simulink model "IEEE_3SG_9bus"  (R2023b)
settings: Solver=ode8  StartTime=0.0  StopTime=20  RelTol=1e-4  EnableMultiTasking=on
PreLoadFcn:
  | ct = 1.083
undefined symbols (not defined in the file): D1, Delta
libraries: spsThreePhaseVIMeasurementLib x12, spsLoadFlowBusLib x9, spsThreePhasePISectionLineLib x6, jailib x3, spsSynchronousMachinepuStandardLib x3, spsThreePhaseTransformerTwoWindingsLib x3, spsDC1AExcitationSystemLib x3, spsPowerPositiveSequenceLib x3, spsThreePhaseBreakerLib x2, spsSequenceAnalyzerLib x1, spsThreePhaseFaultLib x1, spspowerguiLib x1
settings Model: SimulationMode=accelerator  Creator=jp536285  LastModifiedBy=Administrator
settings SolverCC: AlgebraicLoopSolver=TrustRegion  AutoInsertRateTranBlk=on
settings DataIOCC: SaveFormat=Array  SaveOutput=off  SaveTime=off  ReturnWorkspaceOutputs=off
settings OptimizationCC: LifeSpan=inf
settings DebuggingCC: UnderspecifiedInitializationDetection=Classic  MergeDetectMultiDrivingBlocksExec=none  SolverPrmCheckMsg=warning  StateNameClashWarn=warning  SFUnexpectedBacktrackingDiag=warning  SFNoUnconditionalDefaultTransitionDiag=warning  SFExecutionAtInitializationDiag=none  ArithmeticOperatorsInVariantConditions=warning
settings HardwareCC: ProdBitPerPointer=32  ProdBitPerSizeT=32  ProdBitPerPtrDiffT=32  ProdLargestAtomicFloat=None  ProdIntDivRoundTo=Undefined  ProdEndianess=Unspecified  ProdWordSize=32  ProdHWDeviceType=32-bit Generic
settings ModelReferenceCC: PropagateSignalLabelsOutOfModel=off
settings SFSimCC: SimUseLocalCustomCode=off  CustomCodeUndefinedFunction=UseInterfaceOnly
settings RTWCC: RTWUseLocalCustomCode=off
settings CodeAppCC: StateflowObjectComments=on
settings GRTTargetCC: TargetLangStandard=C89/C90 (ANSI)
settings ConfigComp: CovMetricSettings=dw  CovSaveCumulativeToWorkspaceVar=on  CovSaveSingleToWorkspaceVar=on  CovExternalEMLEnable=off
settings SimscapeCC: SimscapeNormalizeSystem=off

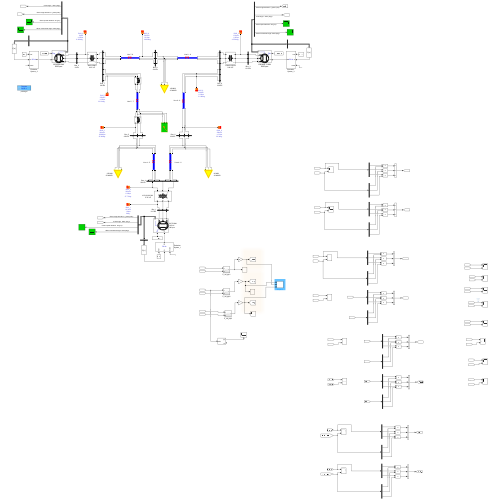
[thumbnail: Simulink's stored preview of the top-level diagram]
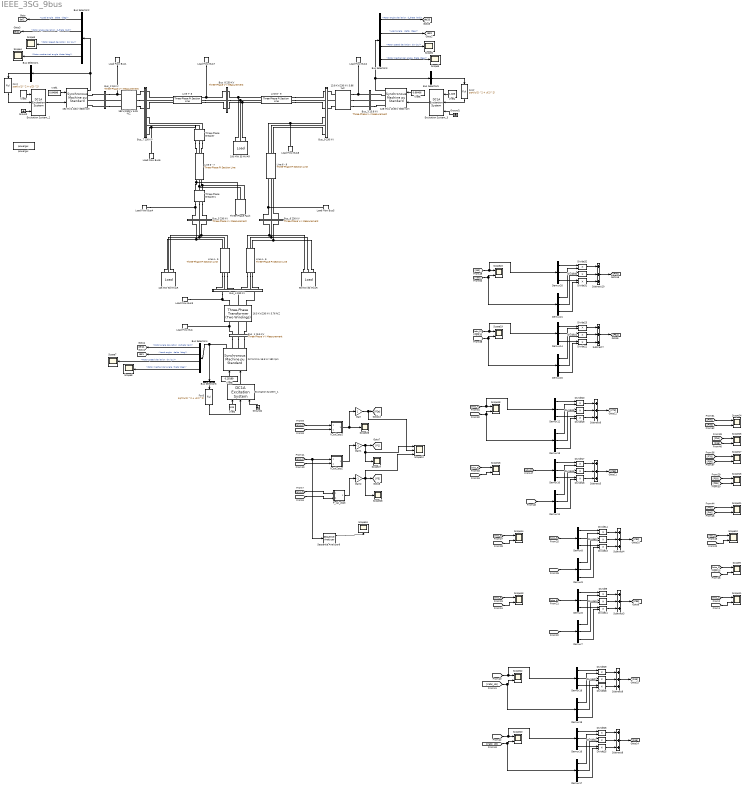
== system IEEE_3SG_9bus ==
  " Line 4 - 6" : spsThreePhasePISectionLineLib/Three-Phase PI Section Line  LConnTagsString=a|b|c  RConnTagsString=A|B|C  Length=100  Frequency=60  Resistances=[ 0.08993 0.224825]  Inductances="[ 1.29e-3  3.22e-3]"  Capacitances=[7.922e-9 4.74e-9]  mask(Three-Phase PI Section Line){}
      mask Display:
      | % This is a new mask on top of the base mask.
      | % Use "View base mask" link below to see the base mask.
      | patch([0.0 0.0 1 1 0.0 0.0 ],[0.4 0.7 0.7 0.4 0.4 0.7],[0 0 1]);
      | patch([0.4 0.4 0.42 0.42],[0.4 0.75 0.75 0.4],[1 0 0]);
      | patch([0.38 0.38 0.57 0.57],[0.7 0.75 0.75 0.7],[1 0 0]);
      | patch([0.53 0.53 0.55 0.55],[0.4 0.75 0.75 0.4],[1 0 0]);
  " Line 6 - 9" : spsThreePhasePISectionLineLib/Three-Phase PI Section Line  LConnTagsString=a|b|c  RConnTagsString=A|B|C  Length=100  Frequency=60  Resistances=[ 0.20631 0.5157]  Inductances="[ 2.38e-3  6.09e-3]"  Capacitances=[17.95e-9 10.55e-9]  mask(Three-Phase PI Section Line){}
      mask Display:
      | % This is a new mask on top of the base mask.
      | % Use "View base mask" link below to see the base mask.
      | patch([0.0 0.0 1 1 0.0 0.0 ],[0.4 0.7 0.7 0.4 0.4 0.7],[0 0 1]);
      | patch([0.4 0.4 0.42 0.42],[0.4 0.75 0.75 0.4],[1 0 0]);
      | patch([0.38 0.38 0.57 0.57],[0.7 0.75 0.75 0.7],[1 0 0]);
      | patch([0.53 0.53 0.55 0.55],[0.4 0.75 0.75 0.4],[1 0 0]);
  100 MW 35 MVAR : jailib/Load  SystemSampleTime=-1  VariantActivationTime=update diagram  AllowFlexibleInterface=on  Latency=0  AutoFrameSizeCalculation=off
      link override Three-Phase Parallel RLC Load: NominalVoltage=(230000)*1.01602  ActivePower=100e6  InductivePower=35e6  LoadType=constant PQ
      settings: SourceProductName=Power Library
  125 MW 50 MVAR : jailib/Load  SystemSampleTime=-1  VariantActivationTime=update diagram  AllowFlexibleInterface=on  Latency=0  AutoFrameSizeCalculation=off
      link override Three-Phase Parallel RLC Load: NominalVoltage=(230000)*0.996183  ActivePower=125e6  InductivePower=50e6  LoadType=constant PQ
      settings: SourceProductName=Power Library
  128 MVA 13.8kV 3600 rpm : spsSynchronousMachinepuStandardLib/Synchronous Machine pu Standard  PresetModel=No  MechanicalLoad=Mechanical power Pm  ShowDetailedParameters=on  RotorType=Round  Units=per unit standard parameters  MeasurementBus=off  NominalParameters="[ 128e6  13.8e3   60 ]"  Reactances1=[ 1.68, 0.23206, 0.19, 1.61, 0.23206, 0.19, 0.314]  Reactances2="[ 1.305, 0.296, 0.252, 0.474,  0.243,  0.18 ]"  dAxisTimeConstants=Open-circuit  qAxisTimeConstants=Open-circuit  TimeConstants1="[ 4.4849  0.0681  0.1  ]"  TimeConstants2=[ 5.89, 0.001,0.6, 0.001 ]  TimeConstants3="[  4.49  0.0681  0.0513  ]"  TimeConstants4=[ 8.0, 0.03, 0.3371, 0.0295 ]  TimeConstants5=[ 1.01, 0.053, 0.1 ]  TimeConstants6=[ 1.3201, 0.023, 1.0, 0.07 ]  TimeConstants7="[  1.01  0.053  0.051266  ]"  TimeConstants8=[ 1.3201, 0.0231, 0.3371, 0.0295 ]  StatorResistance=1e-7  Mechanical="[ 2.35  0 1 ]"  PolePairs=1  InitialConditions=[0 -36.0034 0.653061 0.653061 0.653061 11.785 -108.215 131.785 1.40359]  SetSaturation=off  Saturation=[0.6404,0.7127,0.8441,0.9214,0.9956,1.082,1.19,1.316,1.457;0.7,0.7698,0.8872,0.9466,0.9969,1.046,1.1,1.151,1.201]  LoadFlowParameters=[1 85000000 0 0 0]  TsPowergui=0  TsBlock=-1  IterativeModel=Trapezoidal non iterative  IterativeDiscreteModel=Trapezoidal non iterative  BusType=PV  Pref=85000000  Qref=0  Qmin=-Inf  Qmax=Inf  PLF=0  QLF=0
  13.8 KV/230 KV 5.86 %Z : spsThreePhaseTransformerTwoWindingsLib/Three-Phase Transformer (Two Windings)  Winding1Connection=Delta (D1)  Winding2Connection=Yg  CoreType=Three single-phase transformers  SetSaturation=off  Hysteresis=off  DataFile='hysteresis'  SetInitialFlux=off  Measurements=None  UNITS=pu  NominalPower=[ 100e6 , 60 ]  Winding1=[ 13.8e3 , 1e-6 , 0 ]  Winding2=[ 230e3 , 1e-6, 0.0586 ]  Rm=500  Lm=500  L0=0.5  Saturation=[ 0,0 ; 0.0024,1.2 ; 1.0,1.52 ]  InitialFluxes=[ 0.8 , -0.8 , 0.7 ]  BreakLoop=off  DiscreteSolver=Trapezoidal iterative  DataType=off  TransfoNumber=1
  "16.5 KV/230 KV 5.76 %Z     " : spsThreePhaseTransformerTwoWindingsLib/Three-Phase Transformer (Two Windings)  Winding1Connection=Delta (D1)  Winding2Connection=Yg  CoreType=Three single-phase transformers  SetSaturation=off  Hysteresis=off  DataFile='hysteresis'  SetInitialFlux=off  Measurements=None  UNITS=pu  NominalPower=[ 100e6 , 60 ]  Winding1=[ 16.5e3 , 1e-6, 0 ]  Winding2=[ 230e3 ,1e-6, 0.0576 ]  Rm=500  Lm=500  L0=0.5  Saturation=[ 0,0 ; 0.0024,1.2 ; 1.0,1.52 ]  InitialFluxes=[ 0.8 , -0.8 , 0.7 ]  BreakLoop=off  DiscreteSolver=Trapezoidal iterative  DataType=off  TransfoNumber=1
  18KV/230KV 6.25 %Z : spsThreePhaseTransformerTwoWindingsLib/Three-Phase Transformer (Two Windings)  Winding1Connection=Delta (D1)  Winding2Connection=Yg  CoreType=Three single-phase transformers  SetSaturation=off  Hysteresis=off  DataFile='hysteresis'  SetInitialFlux=off  Measurements=None  UNITS=pu  NominalPower=[ 100e6 , 60 ]  Winding1=[ 18e3 , 1e-6 , 0]  Winding2=[ 230e3 , 1e-6, 0.0625 ]  Rm=500  Lm=500  L0=0.5  Saturation=[ 0,0 ; 0.0024,1.2 ; 1.0,1.52 ]  InitialFluxes=[ 0.8 , -0.8 , 0.7 ]  BreakLoop=off  DiscreteSolver=Trapezoidal iterative  DataType=off  TransfoNumber=1
  192 MVA 18kV 3600 rpm : spsSynchronousMachinepuStandardLib/Synchronous Machine pu Standard  PresetModel=No  MechanicalLoad=Mechanical power Pm  ShowDetailedParameters=on  RotorType=Round  Units=per unit standard parameters  MeasurementBus=off  NominalParameters="[ 192e6  18e3   60 ]"  Reactances1=[ 1.72, 0.23, 0.1728,1.65, 0.23, 0.1728, 0.4224 ]  Reactances2="[ 1.305, 0.296, 0.252, 0.474,  0.243,  0.18 ]"  dAxisTimeConstants=Open-circuit  qAxisTimeConstants=Open-circuit  TimeConstants1="[ 4.4849  0.0681  0.1  ]"  TimeConstants2=[ 6, 0.001, 0.53, 0.001]  TimeConstants3="[  4.49  0.0681  0.0513  ]"  TimeConstants4=[ 8.0, 0.03, 0.3371, 0.0295 ]  TimeConstants5=[ 1.01, 0.053, 0.1 ]  TimeConstants6=[ 1.3201, 0.023, 1.0, 0.07 ]  TimeConstants7="[  1.01  0.053  0.051266  ]"  TimeConstants8=[ 1.3201, 0.0231, 0.3371, 0.0295 ]  StatorResistance=1e-7  Mechanical="[ 3.33  0 1 ]"  PolePairs=1  InitialConditions=[0 -29.1799 0.828949 0.828949 0.828949 6.81655 -113.183 126.817 1.78946]  SetSaturation=off  Saturation=[0.6404,0.7127,0.8441,0.9214,0.9956,1.082,1.19,1.316,1.457;0.7,0.7698,0.8872,0.9466,0.9969,1.046,1.1,1.151,1.201]  LoadFlowParameters=[1 163000000 0 0 0]  TsPowergui=0  TsBlock=-1  IterativeModel=Trapezoidal non iterative  IterativeDiscreteModel=Trapezoidal non iterative  BusType=PV  Pref=163000000  Qref=0  Qmin=-Inf  Qmax=Inf  PLF=0  QLF=0
  247.5 MVA 16.5 kV 180 rpm : spsSynchronousMachinepuStandardLib/Synchronous Machine pu Standard  PresetModel=No  MechanicalLoad=Mechanical power Pm  ShowDetailedParameters=on  RotorType=Salient-pole  Units=per unit standard parameters  MeasurementBus=off  NominalParameters="[ 247.5E6  16500   60 ]"  Reactances1=[ 31 32 33 34 35 36 37 ]  Reactances2=[ 0.361, 0.1504, 0.099, 0.2398, 0.099, 0.062 ]  dAxisTimeConstants=Open-circuit  qAxisTimeConstants=Open-circuit  TimeConstants1=[8.96 0.001 0.001]  TimeConstants2=[]  TimeConstants3=[]  TimeConstants4=[]  TimeConstants5=[ 1.01, 0.053, 0.31 ]  TimeConstants6=[]  TimeConstants7=[]  TimeConstants8=[]  StatorResistance=1e-7  Mechanical=[9.55 0 20]  PolePairs=20  InitialConditions=[0 -86.3839 0.299344 0.299344 0.299344 -20.3492 -140.349 99.6508 1.08182]  SetSaturation=off  Saturation=[0.6404,0.7127,0.8441,0.9214,0.9956,1.082,1.19,1.316,1.457;0.7,0.7698,0.8872,0.9466,0.9969,1.046,1.1,1.151,1.201]  LoadFlowParameters=[2 71000000 0 0]  TsPowergui=0  TsBlock=-1  IterativeModel=Trapezoidal non iterative  IterativeDiscreteModel=Trapezoidal non iterative  BusType=swing  Pref=150000000  Qref=0  Qmin=-Inf  Qmax=Inf  PLF=0  QLF=0
  90 MW 30 MVAR : jailib/Load  SystemSampleTime=-1  VariantActivationTime=update diagram  AllowFlexibleInterface=on  Latency=0  AutoFrameSizeCalculation=off
      link override Three-Phase Parallel RLC Load: NominalVoltage=(230000)*1.01315  ActivePower=90e6  InductivePower=30e6  LoadType=constant PQ
      settings: SourceProductName=Power Library
  Bus Selector1 : BusSelector  OutputSignals="dq0 components.Stator voltage  vq (pu),dq0 components.Stator voltage  vd (pu)"  OutputAsBus=on
  Bus Selector2 : BusSelector  OutputSignals="Load angle   delta  (deg),Mechanical.Rotor angle deviation  d_theta (rad),Mechanical.Rotor speed deviation  dw (pu),Mechanical.Rotor mechanical angle  theta (deg)"
  Bus Selector3 : BusSelector  OutputSignals="Mechanical.Rotor angle deviation  d_theta (rad),Load angle   delta  (deg),Mechanical.Rotor speed deviation  dw (pu),Mechanical.Rotor mechanical angle  theta (deg)"
  Bus Selector4 : BusSelector  OutputSignals="Mechanical.Rotor angle deviation  d_theta (rad),Load angle   delta  (deg),Mechanical.Rotor speed deviation  dw (pu),Mechanical.Rotor mechanical angle  theta (deg)"
  Bus Selector5 : BusSelector  OutputSignals="dq0 components.Stator voltage  vq (pu),dq0 components.Stator voltage  vd (pu)"  OutputAsBus=on
  Bus Selector6 : BusSelector  OutputSignals="dq0 components.Stator voltage  vq (pu),dq0 components.Stator voltage  vd (pu)"  OutputAsBus=on
  Bus_1 16.5 KV : spsThreePhaseVIMeasurementLib/Three-Phase V-I Measurement  VoltageMeasurement=phase-to-phase  SetLabelV=on  LabelV=Vabc_1  Vpu=off  VpuLL=off  CurrentMeasurement=yes  SetLabelI=on  LabelI=Iabc_1  Ipu=off  Pbase=100e6  Vbase=16.5e3  OutputType=Complex  PhasorSimulation=off  PSBequivalent=0
  Bus_2 18 KV : spsThreePhaseVIMeasurementLib/Three-Phase V-I Measurement  VoltageMeasurement=phase-to-phase  SetLabelV=on  LabelV=Vabc_2  Vpu=off  VpuLL=off  CurrentMeasurement=yes  SetLabelI=on  LabelI=Iabc_2  Ipu=off  Pbase=100e6  Vbase=18e3  OutputType=Complex  PhasorSimulation=off  PSBequivalent=0
  Bus_3 13.8 KV : spsThreePhaseVIMeasurementLib/Three-Phase V-I Measurement  VoltageMeasurement=phase-to-phase  SetLabelV=on  LabelV=Vabc_3  Vpu=off  VpuLL=off  CurrentMeasurement=yes  SetLabelI=on  LabelI=Iabc_3  Ipu=off  Pbase=100e6  Vbase=13.8e3  OutputType=Complex  PhasorSimulation=off  PSBequivalent=0
  Bus_4 230 KV : Subsystem
  Bus_5 230 KV : spsThreePhaseVIMeasurementLib/Three-Phase V-I Measurement  VoltageMeasurement=phase-to-ground  SetLabelV=on  LabelV=Vabc_5  Vpu=off  VpuLL=off  CurrentMeasurement=yes  SetLabelI=on  LabelI=Iabc_5  Ipu=off  Pbase=100e6  Vbase=230e3  OutputType=Complex  PhasorSimulation=off  PSBequivalent=0
  Bus_6 230 KV : spsThreePhaseVIMeasurementLib/Three-Phase V-I Measurement  VoltageMeasurement=phase-to-ground  SetLabelV=on  LabelV=Vabc_6  Vpu=off  VpuLL=off  CurrentMeasurement=yes  SetLabelI=on  LabelI=Iabc_6  Ipu=off  Pbase=100e6  Vbase=230e3  OutputType=Complex  PhasorSimulation=off  PSBequivalent=0
  Bus_7 230 KV : Subsystem
  Bus_8 230 KV : spsThreePhaseVIMeasurementLib/Three-Phase V-I Measurement  VoltageMeasurement=phase-to-ground  SetLabelV=on  LabelV=Vabc_8  Vpu=off  VpuLL=off  CurrentMeasurement=yes  SetLabelI=on  LabelI=Iabc_8  Ipu=off  Pbase=100e6  Vbase=230e3  OutputType=Complex  PhasorSimulation=off  PSBequivalent=0
  Bus_9 230 KV : Subsystem
  Demux{6..21} (16 alike) : Demux  Outputs=3
  Divide{9..32} (24 alike) : Product  Inputs=**
  Excitation System_2 : spsDC1AExcitationSystemLib/DC1A Excitation System  Tr=20e-3  KaTa=[20 0.2]  VRminmax=[ -4 4]  KfTf=[0.063 0.35]  TbTc=[0 0]  KeTe=[1 0.314]  Efd12=[3.1 2.3]  SeEfd12=[0.483 0.1394]  v0=[1.025 1.7895]  TsBlock=0
      settings: LibrarySourceBlock=|
      | sps_lib/Electrical Machines/Synchronous Machine Control/DC1A
      | Excitation System
  Excitation System_1 : spsDC1AExcitationSystemLib/DC1A Excitation System  Tr=20e-3  KaTa=[20 0.2]  VRminmax=[ -3 3]  KfTf=[0.063 0.35]  TbTc=[0 0]  KeTe=[1 0.314]  Efd12=[3.1 2.3]  SeEfd12=[0.483 0.1394]  v0=[1.04 1.0818]  TsBlock=0
      settings: LibrarySourceBlock=|
      | sps_lib/Electrical Machines/Synchronous Machine Control/DC1A
      | Excitation System
  Excitation System_3 : spsDC1AExcitationSystemLib/DC1A Excitation System  Tr=20e-3  KaTa=[20 0.2]  VRminmax=[-4 4]  KfTf=[0.063 0.35]  TbTc=[0 0]  KeTe=[1 0.314]  Efd12=[3.1 2.3]  SeEfd12=[0.483 0.1394]  v0=[1.025 1.4036]  TsBlock=0
      settings: LibrarySourceBlock=|
      | sps_lib/Electrical Machines/Synchronous Machine Control/DC1A
      | Excitation System
  Fcn1 : Fcn  Expr=sqrt(u(1)^2 + u(2)^2)
  Fcn2 : Fcn  Expr=sqrt(u(1)^2 + u(2)^2)
  Fcn3 : Fcn  Expr=sqrt(u(1)^2 + u(2)^2)
  Gain : Gain
  Gain1 : Gain  Gain=-1
  Gain2 : Gain  Gain=-1
  Ground : Ground
  Ground1 : Ground
  Ground2 : Ground
  "Line 4 - 5 " : spsThreePhasePISectionLineLib/Three-Phase PI Section Line  LConnTagsString=a|b|c  RConnTagsString=A|B|C  Length=100  Frequency=60  Resistances=[ 0.0529 0.13225]  Inductances="[ 1.192e-3  2.38e-3]"  Capacitances=[8.82e-9 5.188e-9]  mask(Three-Phase PI Section Line){}
      mask Display:
      | % This is a new mask on top of the base mask.
      | % Use "View base mask" link below to see the base mask.
      | patch([0.0 0.0 1 1 0.0 0.0 ],[0.4 0.7 0.7 0.4 0.4 0.7],[0 0 1]);
      | patch([0.4 0.4 0.42 0.42],[0.4 0.75 0.75 0.4],[1 0 0]);
      | patch([0.38 0.38 0.57 0.57],[0.7 0.75 0.75 0.7],[1 0 0]);
      | patch([0.53 0.53 0.55 0.55],[0.4 0.75 0.75 0.4],[1 0 0]);
  "Line 5 - 7 " : spsThreePhasePISectionLineLib/Three-Phase PI Section Line  LConnTagsString=a|b|c  RConnTagsString=A|B|C  Length=100  Frequency=60  Resistances=[ 0.16928 0.4232]  Inductances="[ 2.259e-3  5.64e-3]"  Capacitances=[15.34e-9 9.025e-9]  mask(Three-Phase PI Section Line){}
      mask Display:
      | % This is a new mask on top of the base mask.
      | % Use "View base mask" link below to see the base mask.
      | patch([0.0 0.0 1 1 0.0 0.0 ],[0.4 0.7 0.7 0.4 0.4 0.7],[0 0 1]);
      | patch([0.4 0.4 0.42 0.42],[0.4 0.75 0.75 0.4],[1 0 0]);
      | patch([0.38 0.38 0.57 0.57],[0.7 0.75 0.75 0.7],[1 0 0]);
      | patch([0.53 0.53 0.55 0.55],[0.4 0.75 0.75 0.4],[1 0 0]);
  Line 7- 8 : spsThreePhasePISectionLineLib/Three-Phase PI Section Line  LConnTagsString=a|b|c  RConnTagsString=A|B|C  Length=100  Frequency=60  Resistances=[0.044965 0.11241]  Inductances="[ 1.01e-3  2.02e-3]"  Capacitances=[7.471e-9 4.394e-9]  mask(Three-Phase PI Section Line){}
      mask Display:
      | % This is a new mask on top of the base mask.
      | % Use "View base mask" link below to see the base mask.
      | patch([0.0 0.0 1 1 0.0 0.0 ],[0.4 0.7 0.7 0.4 0.4 0.7],[0 0 1]);
      | patch([0.4 0.4 0.42 0.42],[0.4 0.75 0.75 0.4],[1 0 0]);
      | patch([0.38 0.38 0.57 0.57],[0.7 0.75 0.75 0.7],[1 0 0]);
      | patch([0.53 0.53 0.55 0.55],[0.4 0.75 0.75 0.4],[1 0 0]);
  Line 8 - 9 : spsThreePhasePISectionLineLib/Three-Phase PI Section Line  LConnTagsString=a|b|c  RConnTagsString=A|B|C  Length=100  Frequency=60  Resistances=[ 0.062951 0.15737]  Inductances="[ 1.414e-3  3.53e-3]"  Capacitances=[10.47e-9 6.15e-9]  mask(Three-Phase PI Section Line){}
      mask Display:
      | % This is a new mask on top of the base mask.
      | % Use "View base mask" link below to see the base mask.
      | patch([0.0 0.0 1 1 0.0 0.0 ],[0.4 0.7 0.7 0.4 0.4 0.7],[0 0 1]);
      | patch([0.4 0.4 0.42 0.42],[0.4 0.75 0.75 0.4],[1 0 0]);
      | patch([0.38 0.38 0.57 0.57],[0.7 0.75 0.75 0.7],[1 0 0]);
      | patch([0.53 0.53 0.55 0.55],[0.4 0.75 0.75 0.4],[1 0 0]);
  Load Flow Bus : spsLoadFlowBusLib/Load Flow Bus  LConnTagsString=a  Phases=single  Connectors=on one side  ID=BUS_1  Vbase=16.5e3  Vref=1.04  Vangle=0  VLF=1.04  VLFb=1  VLFc=1  angleLF=0  angleLFb=0  angleLFc=0
      settings: AttributesFormatString=%<ID>\n%<Vbase>V\n%<VLF>pu\n%<angleLF>deg.
  Load Flow Bus1 : spsLoadFlowBusLib/Load Flow Bus  LConnTagsString=a  Phases=single  Connectors=on one side  ID=BUS_2  Vbase=18e3  Vref=1.025  Vangle=0  VLF=1.025  VLFb=1  VLFc=1  angleLF=9.166  angleLFb=0  angleLFc=0
      settings: AttributesFormatString=%<ID>\n%<Vbase>V\n%<VLF>pu\n%<angleLF>deg.
  Load Flow Bus2 : spsLoadFlowBusLib/Load Flow Bus  LConnTagsString=a  Phases=single  Connectors=on one side  ID=BUS_3  Vbase=13.8e3  Vref=1.025  Vangle=0  VLF=1.025  VLFb=1  VLFc=1  angleLF=4.553  angleLFb=0  angleLFc=0
      settings: AttributesFormatString=%<ID>\n%<Vbase>V\n%<VLF>pu\n%<angleLF>deg.
  Load Flow Bus3 : spsLoadFlowBusLib/Load Flow Bus  LConnTagsString=a  Phases=single  Connectors=on one side  ID=BUS_4  Vbase=230e3  Vref=1  Vangle=0  VLF=1.026  VLFb=1  VLFc=1  angleLF=27.77  angleLFb=0  angleLFc=0
      settings: AttributesFormatString=%<ID>\n%<Vbase>V\n%<VLF>pu\n%<angleLF>deg.
  Load Flow Bus4 : spsLoadFlowBusLib/Load Flow Bus  LConnTagsString=a  Phases=single  Connectors=on one side  ID=BUS_5  Vbase=230e3  Vref=1  Vangle=0  VLF=0.9962  VLFb=1  VLFc=1  angleLF=25.99  angleLFb=0  angleLFc=0
      settings: AttributesFormatString=%<ID>\n%<Vbase>V\n%<VLF>pu\n%<angleLF>deg.
  Load Flow Bus5 : spsLoadFlowBusLib/Load Flow Bus  LConnTagsString=a  Phases=single  Connectors=on one side  ID=BUS_6  Vbase=230e3  Vref=1  Vangle=0  VLF=1.013  VLFb=1  VLFc=1  angleLF=26.3  angleLFb=0  angleLFc=0
      settings: AttributesFormatString=%<ID>\n%<Vbase>V\n%<VLF>pu\n%<angleLF>deg.
  Load Flow Bus6 : spsLoadFlowBusLib/Load Flow Bus  LConnTagsString=a  Phases=single  Connectors=on one side  ID=BUS_7  Vbase=230e3  Vref=1  Vangle=0  VLF=1.026  VLFb=1  VLFc=1  angleLF=33.61  angleLFb=0  angleLFc=0
      settings: AttributesFormatString=%<ID>\n%<Vbase>V\n%<VLF>pu\n%<angleLF>deg.
  Load Flow Bus7 : spsLoadFlowBusLib/Load Flow Bus  LConnTagsString=a  Phases=single  Connectors=on one side  ID=BUS_8  Vbase=230e3  Vref=1  Vangle=0  VLF=1.016  VLFb=1  VLFc=1  angleLF=30.63  angleLFb=0  angleLFc=0
      settings: AttributesFormatString=%<ID>\n%<Vbase>V\n%<VLF>pu\n%<angleLF>deg.
  Load Flow Bus8 : spsLoadFlowBusLib/Load Flow Bus  LConnTagsString=a  Phases=single  Connectors=on one side  ID=BUS_9  Vbase=230e3  Vref=1  Vangle=0  VLF=1.032  VLFb=1  VLFc=1  angleLF=31.86  angleLFb=0  angleLFc=0
      settings: AttributesFormatString=%<ID>\n%<Vbase>V\n%<VLF>pu\n%<angleLF>deg.
  P_cal_ptp1 : Subsystem
  P_cal_ptp2 : Subsystem
  P_cal_ptp3 : Subsystem
  Scope{9..11,13..25} (16 alike) : Scope  NumInputPorts=2
  Scope12 : Scope  NumInputPorts=3
  Scope{2..5,7..8,26..28,34} (10 alike) : Scope
  Sequence Analyzer9 : spsSequenceAnalyzerLib/Sequence Analyzer  Freq=60  n=1  seq=Positive  InInit=[1, 0]  Ts=0
      settings: LibrarySourceBlock=sps_lib/Sensors and Measurements/Sequence Analyzer
  Subtract{3..10} (8 alike) : Sum  Inputs=+++
  Three-Phase Breaker : spsThreePhaseBreakerLib/Three-Phase Breaker  InitialState=closed  SwitchA=on  SwitchB=on  SwitchC=on  SwitchTimes=10+ct  External=off  BreakerResistance=0.001  SnubberResistance=1e7  SnubberCapacitance=inf  Measurements=None
  Three-Phase Breaker1 : spsThreePhaseBreakerLib/Three-Phase Breaker  InitialState=closed  SwitchA=on  SwitchB=on  SwitchC=on  SwitchTimes=10+ct  External=off  BreakerResistance=0.001  SnubberResistance=1e7  SnubberCapacitance=inf  Measurements=None
  Three-Phase Fault : spsThreePhaseFaultLib/Three-Phase Fault  InitialStates=0  FaultA=on  FaultB=on  FaultC=on  GroundFault=off  SwitchTimes=[ 10 10+ct]  External=off  SwitchStatus=NaN  FaultResistance=0.001  GroundResistance=0.001  SnubberResistance=1e6  SnubberCapacitance=inf  Measurements=None
  Vref1 : Constant  Value=0.84896
  Vref2 : Constant  Value=1.04
  Vref3 : Constant  Value=1.025
  Vref4 : Constant  Value=1.025
  Vref5 : Constant  Value=0.66406
  Vref8 : Constant  Value=0.29189
  powergui : spspowerguiLib/powergui  Priority=1  SimulationMode=Discrete  SampleTime=5e-5  frequency=60  Iterations=50  frequencyindice=60  Pbase=10e7  ErrMax=1e-05  UnitsV=kV  UnitsW=MW  buscounter=0  FunctionMessages=off  echomessages=off  EnableUseOfTLC=off  CurrentSourceSwitches=off  DisableSnubberDevices=off  DisableRonSwitches=off  DisableVfSwitches=off  DisplayEquations=off  AutomaticDiscreteSolvers=off  SolverType=Backward Euler  Interpol=off  ExternalGateDelay=off  methode=off  Ts=0  x0status=blocks  SPID=off  SwTol=0  HookPort=off  NonlinearTolerance=1e-4  nMaxIteration=100  ContinueOnMaxIteration=off  RestoreLinks=warning  ResistiveCurrentMeasurement=off  Frange=[0:2:500]  Ylog=off  Xlog=on  ShowGrid=off  save=off  variable=ZData  structure=0  ZoomFFT=off  StartTime=0.0  cycles=1  DisplayStyle=1  fundamental=60  FreqAxis=off  MaxFrequency=1000  frequencyindicesteady=1  RmsSteady=1  display=off
  tag scope: del11=global, del1=global, del22=global, del2=global, del33=global, del3=global
  wires:
  Vref5/1 -> 128 MVA 13.8kV 3600 rpm/1
  Excitation System_3/1 -> 128 MVA 13.8kV 3600 rpm/2
  192 MVA 18kV 3600 rpm/1 -> Bus Selector2/1, Bus Selector1/1
  Bus Selector2/1 -> [del2]  "<Load angle   delta  (deg)>"
  Bus Selector3/2 -> [del3]  "<Load angle   delta  (deg)>"
  128 MVA 13.8kV 3600 rpm/1 -> Bus Selector3/1, Bus Selector5/1
  247.5 MVA 16.5 kV 180 rpm/1 -> Bus Selector4/1, Bus Selector6/1
  Vref8/1 -> 247.5 MVA 16.5 kV 180 rpm/1
  Excitation System_1/1 -> 247.5 MVA 16.5 kV 180 rpm/2
  Bus Selector4/2 -> [del1]  "<Load angle   delta  (deg)>"
  Vref3/1 -> Excitation System_2/1
  Ground/1 -> Excitation System_2/3
  Vref4/1 -> Excitation System_3/1
  Ground1/1 -> Excitation System_3/3
  Vref2/1 -> Excitation System_1/1
  Bus Selector2/2 -> [del22]  "<Rotor angle deviation  d_theta (rad)>"
  Bus Selector4/1 -> [del11]  "<Rotor angle deviation  d_theta (rad)>"
  Bus Selector3/1 -> [del33]  "<Rotor angle deviation  d_theta (rad)>"
  Bus Selector2/3 -> Scope3/1  "<Rotor speed deviation  dw (pu)>"
  Vref1/1 -> 192 MVA 18kV 3600 rpm/1
  Bus Selector2/4 -> Scope4/1  "<Rotor mechanical angle  theta (deg)>"
  Bus Selector3/3 -> Scope2/1  "<Rotor speed deviation  dw (pu)>"
  Bus Selector3/4 -> Scope5/1  "<Rotor mechanical angle  theta (deg)>"
  Bus Selector4/3 -> Scope7/1  "<Rotor speed deviation  dw (pu)>"
  Bus Selector4/4 -> Scope8/1  "<Rotor mechanical angle  theta (deg)>"
  Bus Selector1/1 -> Fcn1/1
  Fcn1/1 -> Excitation System_2/2
  Excitation System_2/1 -> 192 MVA 18kV 3600 rpm/2
  Bus Selector5/1 -> Fcn2/1
  Fcn2/1 -> Excitation System_3/2
  Ground2/1 -> Excitation System_1/3
  Bus Selector6/1 -> Fcn3/1
  Fcn3/1 -> Excitation System_1/2
  [Iabc_2] -> Scope9/1
  Subtract8/1 -> [P46]
  [Vabc_5] -> Demux15/1, Scope19/2
  [Iabc_1] -> Scope11/1
  Demux19/1 -> Divide29/2
  Demux15/2 -> Divide21/2
  Subtract5/1 -> [P98]
  Demux14/3 -> Divide22/1
  Divide31/1 -> Subtract10/3
  Divide19/1 -> Subtract6/3
  [P78] -> Scope17/1
  [P96] -> Scope15/2
  Subtract4/1 -> [P93]
  [P93] -> Scope15/1
  Divide15/1 -> Subtract5/2
  Subtract7/1 -> [P54]
  Subtract3/1 -> [P96]
  [Vabc_8] -> Scope16/2
  Divide29/1 -> Subtract9/1
  Demux10/3 -> Divide16/1
  Demux17/1 -> Divide26/2
  [Vabc_3] -> Scope10/2
  [P98] -> Scope17/2
  Divide28/1 -> Subtract9/3
  Demux20/2 -> Divide30/1
  [Vabc_2] -> Scope9/2
  Demux20/1 -> Divide32/1
  Demux7/3 -> Divide11/2
  [Vabc_8] -> Demux11/1
  Divide14/1 -> Subtract4/1
  Subtract10/1 -> [P75]
  Divide12/1 -> Subtract4/2
  [Vabc_1] -> Scope11/2
  Demux10/1 -> Divide17/1
  Demux16/1 -> Divide26/1
  [P45] -> Scope25/2
  Demux16/2 -> Divide24/1
  Demux19/3 -> Divide28/2
  [P46] -> Scope21/2
  Divide25/1 -> Subtract8/3
  [Iabc_6] -> Scope13/1
  [P54] -> Scope25/1
  [Iabc_6] -> Demux6/1
  [Iabc_3] -> Scope10/1
  Demux11/3 -> Divide16/2
  Demux17/3 -> Divide25/2
  Demux19/2 -> Divide27/2
  Demux18/2 -> Divide27/1
  Demux11/2 -> Divide15/2
  [Iabc_9] -> Scope14/1
  [Vabc_45] -> Scope22/2, Demux19/1
  Divide13/1 -> Subtract4/3
  Demux6/1 -> Divide9/1
  Demux14/2 -> Divide21/1
  Demux13/1 -> Divide20/2
  Demux16/3 -> Divide25/1
  Divide27/1 -> Subtract9/2
  Divide9/1 -> Subtract3/1
  [Iabc_45] -> Demux18/1, Scope22/1
  Demux9/3 -> Divide13/2
  Divide11/1 -> Subtract3/3
  Demux12/3 -> Divide19/1
  [Vabc_46] -> Demux17/1, Scope20/2
  [Vabc_6] -> Scope13/2
  Demux8/3 -> Divide13/1
  [Iabc_8] -> Scope16/1
  [Vab] -> Demux21/1, Scope23/2
  Demux13/2 -> Divide18/2
  Demux10/2 -> Divide15/1
  [Iabc_46] -> Demux16/1, Scope20/1
  [Vabc_9] -> Scope14/2
  Divide16/1 -> Subtract5/3
  Demux13/3 -> Divide19/2
  Divide30/1 -> Subtract10/2
  [Iabc_7] -> Demux12/1, Scope18/1
  [Vabc_7] -> Demux13/1, Scope18/2
  Demux8/2 -> Divide12/1
  Demux6/2 -> Divide10/1
  Demux9/2 -> Divide12/2
  Demux7/1 -> Divide9/2
  [Vabc_9] -> Demux9/1
  Divide18/1 -> Subtract6/2
  Demux11/1 -> Divide17/2
  [Iabc_9] -> Demux8/1
  Subtract6/1 -> [P78]
  Divide24/1 -> Subtract8/2
  Demux8/1 -> Divide14/1
  Demux15/3 -> Divide22/2
  Demux9/1 -> Divide14/2
  Demux12/1 -> Divide20/1
  Divide32/1 -> Subtract10/1
  Divide22/1 -> Subtract7/3
  [Vabc_6] -> Demux7/1
  Demux17/2 -> Divide24/2
  Divide20/1 -> Subtract6/1
  Demux21/3 -> Divide31/2
  Demux14/1 -> Divide23/1
  Demux21/2 -> Divide30/2
  Demux20/3 -> Divide31/1
  Divide10/1 -> Subtract3/2
  [Iab] -> Demux20/1, Scope23/1
  Demux15/1 -> Divide23/2
  [Iabc_5] -> Demux14/1, Scope19/1
  Divide17/1 -> Subtract5/1
  [P45] -> Scope21/1
  Demux7/2 -> Divide10/2
  [P75] -> Scope24/1
  [P78] -> Scope24/2
  Subtract9/1 -> [P45]
  Demux18/1 -> Divide29/1
  Demux12/2 -> Divide18/1
  Divide23/1 -> Subtract7/1
  Demux6/3 -> Divide11/1
  Divide21/1 -> Subtract7/2
  Divide26/1 -> Subtract8/1
  Demux21/1 -> Divide32/2
  Demux18/3 -> Divide28/1
  [Iabc_8] -> Demux10/1
  P_cal_ptp1/1(Out1) -> Gain/1, Scope26/1
  Gain/1 -> Scope12/2, [P2e]
  Gain1/1 -> Scope12/1, Scope27/1, [P1]
  P_cal_ptp2/1(Out1) -> Gain1/1
  [Iabc_2] -> P_cal_ptp1/1(In1)
  P_cal_ptp3/1(Out1) -> Gain2/1
  [Iabc_1] -> P_cal_ptp2/1(In1), Sequence Analyzer9/1
  Sequence Analyzer9/1 -> Scope34/1
  Gain2/1 -> Scope12/3, Scope28/1, [P3]
  [Iabc_3] -> P_cal_ptp3/1(In1)
  [Vabc_3] -> P_cal_ptp3/2(In2)
  [Vabc_2] -> P_cal_ptp1/2(In2)
  [Vabc_1] -> P_cal_ptp2/2(In2)
  connections:
  Bus_2 18 KV/LConn2 -- 192 MVA 18kV 3600 rpm/RConn2
  18KV/230KV 6.25 %Z/LConn2 -- Bus_2 18 KV/RConn2
  18KV/230KV 6.25 %Z/RConn2 -- Bus_7 230 KV/LConn2
  Bus_2 18 KV/RConn1 -- Load Flow Bus1/LConn1 -- 18KV/230KV 6.25 %Z/LConn1
  Bus_2 18 KV/RConn3 -- 18KV/230KV 6.25 %Z/LConn3
  Bus_7 230 KV/LConn1 -- 18KV/230KV 6.25 %Z/RConn1
  18KV/230KV 6.25 %Z/RConn3 -- Bus_7 230 KV/LConn3
  13.8 KV/230 KV 5.86 %Z/LConn1 -- Bus_3 13.8 KV/LConn1 -- Load Flow Bus2/LConn1
  13.8 KV/230 KV 5.86 %Z/LConn2 -- Bus_3 13.8 KV/LConn2
  13.8 KV/230 KV 5.86 %Z/LConn3 -- Bus_3 13.8 KV/LConn3
  Bus_1 16.5 KV/RConn1 -- 247.5 MVA 16.5 kV 180 rpm/RConn1
  Bus_1 16.5 KV/RConn2 -- 247.5 MVA 16.5 kV 180 rpm/RConn2
  Bus_1 16.5 KV/RConn3 -- 247.5 MVA 16.5 kV 180 rpm/RConn3
  Bus_1 16.5 KV/LConn3 -- "16.5 KV/230 KV 5.76 %Z     "/LConn3
  Bus_1 16.5 KV/LConn2 -- "16.5 KV/230 KV 5.76 %Z     "/LConn2
  13.8 KV/230 KV 5.86 %Z/RConn1 -- Bus_9 230 KV/RConn1
  13.8 KV/230 KV 5.86 %Z/RConn2 -- Bus_9 230 KV/RConn2
  13.8 KV/230 KV 5.86 %Z/RConn3 -- Bus_9 230 KV/RConn3
  Bus_4 230 KV/LConn1 -- "16.5 KV/230 KV 5.76 %Z     "/RConn1 -- Load Flow Bus3/LConn1
  Bus_4 230 KV/LConn2 -- "16.5 KV/230 KV 5.76 %Z     "/RConn2
  Line 8 - 9/LConn1 -- Bus_8 230 KV/LConn1 -- 100 MW 35 MVAR/LConn1
  Line 8 - 9/LConn2 -- 100 MW 35 MVAR/LConn2 -- Bus_8 230 KV/LConn2
  Line 8 - 9/LConn3 -- 100 MW 35 MVAR/LConn3 -- Bus_8 230 KV/LConn3
  "16.5 KV/230 KV 5.76 %Z     "/RConn3 -- Bus_4 230 KV/LConn3
  "Line 4 - 5 "/LConn1 -- 125 MW 50 MVAR/LConn1 -- Bus_5 230 KV/RConn1
  "Line 4 - 5 "/LConn2 -- 125 MW 50 MVAR/LConn2 -- Bus_5 230 KV/RConn2
  "Line 4 - 5 "/LConn3 -- 125 MW 50 MVAR/LConn3 -- Bus_5 230 KV/RConn3
  " Line 4 - 6"/LConn1 -- 90 MW 30 MVAR/LConn1 -- Bus_6 230 KV/RConn1
  " Line 4 - 6"/LConn2 -- 90 MW 30 MVAR/LConn2 -- Bus_6 230 KV/RConn2
  " Line 4 - 6"/LConn3 -- 90 MW 30 MVAR/LConn3 -- Bus_6 230 KV/RConn3
  Line 7- 8/LConn1 -- Bus_7 230 KV/RConn1
  Line 7- 8/LConn2 -- Bus_7 230 KV/RConn2
  Bus_7 230 KV/RConn3 -- Line 7- 8/LConn3
  Bus_8 230 KV/RConn1 -- Line 7- 8/RConn1 -- Load Flow Bus7/LConn1
  Line 7- 8/RConn2 -- Bus_8 230 KV/RConn2
  Line 7- 8/RConn3 -- Bus_8 230 KV/RConn3
  Line 8 - 9/RConn2 -- Bus_9 230 KV/LConn2
  Line 8 - 9/RConn1 -- Bus_9 230 KV/LConn1
  Line 8 - 9/RConn3 -- Bus_9 230 KV/LConn3
  Bus_7 230 KV/RConn6 -- Three-Phase Breaker/LConn1 -- Load Flow Bus6/LConn1
  " Line 6 - 9"/RConn1 -- Load Flow Bus8/LConn1 -- Bus_9 230 KV/LConn4
  Bus_9 230 KV/LConn5 -- " Line 6 - 9"/RConn2
  Bus_6 230 KV/LConn1 -- " Line 6 - 9"/LConn1 -- Load Flow Bus5/LConn1
  Bus_6 230 KV/LConn2 -- " Line 6 - 9"/LConn2
  Bus_6 230 KV/LConn3 -- " Line 6 - 9"/LConn3
  " Line 6 - 9"/RConn3 -- Bus_9 230 KV/LConn6
  "Line 4 - 5 "/RConn2 -- Bus_4 230 KV/RConn2
  "Line 4 - 5 "/RConn1 -- Bus_4 230 KV/RConn1
  "Line 4 - 5 "/RConn3 -- Bus_4 230 KV/RConn3
  " Line 4 - 6"/RConn2 -- Bus_4 230 KV/RConn5
  " Line 4 - 6"/RConn1 -- Bus_4 230 KV/RConn4
  " Line 4 - 6"/RConn3 -- Bus_4 230 KV/RConn6
  128 MVA 13.8kV 3600 rpm/RConn1 -- Bus_3 13.8 KV/RConn1
  128 MVA 13.8kV 3600 rpm/RConn2 -- Bus_3 13.8 KV/RConn2
  Bus_3 13.8 KV/RConn3 -- 128 MVA 13.8kV 3600 rpm/RConn3
  Bus_2 18 KV/LConn3 -- 192 MVA 18kV 3600 rpm/RConn3
  Bus_2 18 KV/LConn1 -- 192 MVA 18kV 3600 rpm/RConn1
  Bus_1 16.5 KV/LConn1 -- Load Flow Bus/LConn1 -- "16.5 KV/230 KV 5.76 %Z     "/LConn1
  Three-Phase Breaker/RConn2 -- "Line 5 - 7 "/LConn2
  Three-Phase Breaker/RConn1 -- "Line 5 - 7 "/LConn1
  Three-Phase Breaker/RConn3 -- "Line 5 - 7 "/LConn3
  Three-Phase Breaker/LConn2 -- Bus_7 230 KV/RConn5
  Three-Phase Breaker/LConn3 -- Bus_7 230 KV/RConn4
  Three-Phase Breaker1/LConn2 -- "Line 5 - 7 "/RConn2 -- Three-Phase Fault/LConn2
  Three-Phase Breaker1/RConn2 -- Bus_5 230 KV/LConn2
  Three-Phase Breaker1/LConn1 -- Three-Phase Fault/LConn1 -- "Line 5 - 7 "/RConn1
  Three-Phase Breaker1/LConn3 -- Three-Phase Fault/LConn3 -- "Line 5 - 7 "/RConn3
  Three-Phase Breaker1/RConn3 -- Bus_5 230 KV/LConn3
  Three-Phase Breaker1/RConn1 -- Load Flow Bus4/LConn1 -- Bus_5 230 KV/LConn1

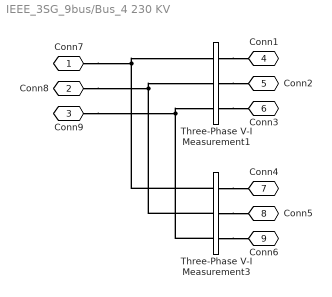
== system IEEE_3SG_9bus/Bus_4 230 KV ==
  Three-Phase V-I Measurement1 : spsThreePhaseVIMeasurementLib/Three-Phase V-I Measurement  VoltageMeasurement=phase-to-ground  SetLabelV=on  LabelV=Vabc_45  Vpu=off  VpuLL=off  CurrentMeasurement=yes  SetLabelI=on  LabelI=Iabc_45  Ipu=off  Pbase=100e6  Vbase=230e3  OutputType=Complex  PhasorSimulation=off  PSBequivalent=0
  Three-Phase V-I Measurement3 : spsThreePhaseVIMeasurementLib/Three-Phase V-I Measurement  VoltageMeasurement=phase-to-ground  SetLabelV=on  LabelV=Vabc_46  Vpu=off  VpuLL=off  CurrentMeasurement=yes  SetLabelI=on  LabelI=Iabc_46  Ipu=off  Pbase=100e6  Vbase=230e3  OutputType=Complex  PhasorSimulation=off  PSBequivalent=0
  Conn7 : PMIOPort  Side=Left
  Conn8 : PMIOPort  Port=2  Side=Left
  Conn9 : PMIOPort  Port=3  Side=Left
  Conn1 : PMIOPort  Port=4  Side=Right
  Conn2 : PMIOPort  Port=5  Side=Right
  Conn3 : PMIOPort  Port=6  Side=Right
  Conn4 : PMIOPort  Port=7  Side=Right
  Conn5 : PMIOPort  Port=8  Side=Right
  Conn6 : PMIOPort  Port=9  Side=Right
  connections:
  Three-Phase V-I Measurement3/LConn3 -- Conn9/RConn1 -- Three-Phase V-I Measurement1/LConn3
  Three-Phase V-I Measurement3/LConn2 -- Conn8/RConn1 -- Three-Phase V-I Measurement1/LConn2
  Three-Phase V-I Measurement3/LConn1 -- Conn7/RConn1 -- Three-Phase V-I Measurement1/LConn1
  Three-Phase V-I Measurement3/RConn3 -- Conn6/RConn1
  Three-Phase V-I Measurement1/RConn3 -- Conn3/RConn1
  Three-Phase V-I Measurement1/RConn1 -- Conn1/RConn1
  Three-Phase V-I Measurement1/RConn2 -- Conn2/RConn1
  Three-Phase V-I Measurement3/RConn1 -- Conn4/RConn1
  Three-Phase V-I Measurement3/RConn2 -- Conn5/RConn1

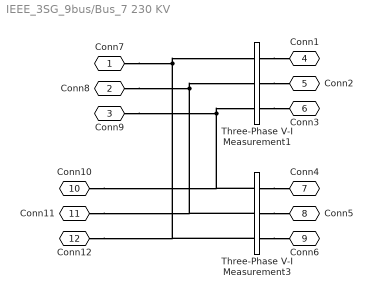
== system IEEE_3SG_9bus/Bus_7 230 KV ==
  Three-Phase V-I Measurement1 : spsThreePhaseVIMeasurementLib/Three-Phase V-I Measurement  VoltageMeasurement=phase-to-ground  SetLabelV=on  LabelV=Vabc_7  Vpu=off  VpuLL=off  CurrentMeasurement=yes  SetLabelI=on  LabelI=Iabc_7  Ipu=off  Pbase=100e6  Vbase=230e3  OutputType=Complex  PhasorSimulation=off  PSBequivalent=0
  Three-Phase V-I Measurement3 : spsThreePhaseVIMeasurementLib/Three-Phase V-I Measurement  VoltageMeasurement=phase-to-ground  SetLabelV=on  LabelV=Vab  Vpu=off  VpuLL=off  CurrentMeasurement=yes  SetLabelI=on  LabelI=Iab  Ipu=off  Pbase=100e6  Vbase=230e3  OutputType=Complex  PhasorSimulation=off  PSBequivalent=0
  Conn7 : PMIOPort  Side=Left
  Conn8 : PMIOPort  Port=2  Side=Left
  Conn9 : PMIOPort  Port=3  Side=Left
  Conn1 : PMIOPort  Port=4  Side=Right
  Conn2 : PMIOPort  Port=5  Side=Right
  Conn3 : PMIOPort  Port=6  Side=Right
  Conn4 : PMIOPort  Port=7  Side=Right
  Conn5 : PMIOPort  Port=8  Side=Right
  Conn6 : PMIOPort  Port=9  Side=Right
  Conn10 : PMIOPort  Port=10  Side=Left
  Conn11 : PMIOPort  Port=11  Side=Left
  Conn12 : PMIOPort  Port=12  Side=Left
  connections:
  Three-Phase V-I Measurement3/RConn2 -- Conn5/RConn1
  Three-Phase V-I Measurement3/RConn1 -- Conn4/RConn1
  Three-Phase V-I Measurement1/RConn2 -- Conn2/RConn1
  Three-Phase V-I Measurement1/RConn1 -- Conn1/RConn1
  Three-Phase V-I Measurement1/RConn3 -- Conn3/RConn1
  Three-Phase V-I Measurement3/RConn3 -- Conn6/RConn1
  Conn7/RConn1 -- Three-Phase V-I Measurement3/LConn3 -- Conn12/RConn1 -- Three-Phase V-I Measurement1/LConn1
  Conn8/RConn1 -- Three-Phase V-I Measurement3/LConn2 -- Conn11/RConn1 -- Three-Phase V-I Measurement1/LConn2
  Conn9/RConn1 -- Conn10/RConn1 -- Three-Phase V-I Measurement3/LConn1 -- Three-Phase V-I Measurement1/LConn3

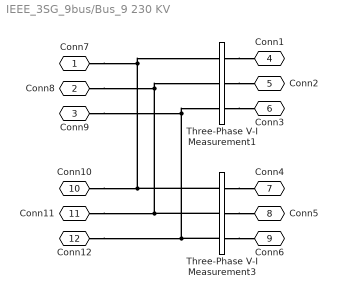
== system IEEE_3SG_9bus/Bus_9 230 KV ==
  Three-Phase V-I Measurement1 : spsThreePhaseVIMeasurementLib/Three-Phase V-I Measurement  VoltageMeasurement=phase-to-ground  SetLabelV=on  LabelV=Vabc_9  Vpu=off  VpuLL=off  CurrentMeasurement=yes  SetLabelI=on  LabelI=Iabc_9  Ipu=off  Pbase=100e6  Vbase=230e3  OutputType=Complex  PhasorSimulation=off  PSBequivalent=0
  Three-Phase V-I Measurement3 : spsThreePhaseVIMeasurementLib/Three-Phase V-I Measurement  VoltageMeasurement=phase-to-ground  SetLabelV=on  LabelV=Vabc  Vpu=off  VpuLL=off  CurrentMeasurement=yes  SetLabelI=on  LabelI=Iabc  Ipu=off  Pbase=100e6  Vbase=230e3  OutputType=Complex  PhasorSimulation=off  PSBequivalent=0
  Conn7 : PMIOPort  Side=Left
  Conn8 : PMIOPort  Port=2  Side=Left
  Conn9 : PMIOPort  Port=3  Side=Left
  Conn1 : PMIOPort  Port=4  Side=Right
  Conn2 : PMIOPort  Port=5  Side=Right
  Conn3 : PMIOPort  Port=6  Side=Right
  Conn4 : PMIOPort  Port=7  Side=Right
  Conn5 : PMIOPort  Port=8  Side=Right
  Conn6 : PMIOPort  Port=9  Side=Right
  Conn10 : PMIOPort  Port=10  Side=Left
  Conn11 : PMIOPort  Port=11  Side=Left
  Conn12 : PMIOPort  Port=12  Side=Left
  connections:
  Conn12/RConn1 -- Three-Phase V-I Measurement3/LConn3 -- Conn9/RConn1 -- Three-Phase V-I Measurement1/LConn3
  Conn11/RConn1 -- Three-Phase V-I Measurement3/LConn2 -- Conn8/RConn1 -- Three-Phase V-I Measurement1/LConn2
  Conn10/RConn1 -- Three-Phase V-I Measurement3/LConn1 -- Conn7/RConn1 -- Three-Phase V-I Measurement1/LConn1
  Three-Phase V-I Measurement3/RConn3 -- Conn6/RConn1
  Three-Phase V-I Measurement1/RConn3 -- Conn3/RConn1
  Three-Phase V-I Measurement1/RConn1 -- Conn1/RConn1
  Three-Phase V-I Measurement1/RConn2 -- Conn2/RConn1
  Three-Phase V-I Measurement3/RConn1 -- Conn4/RConn1
  Three-Phase V-I Measurement3/RConn2 -- Conn5/RConn1

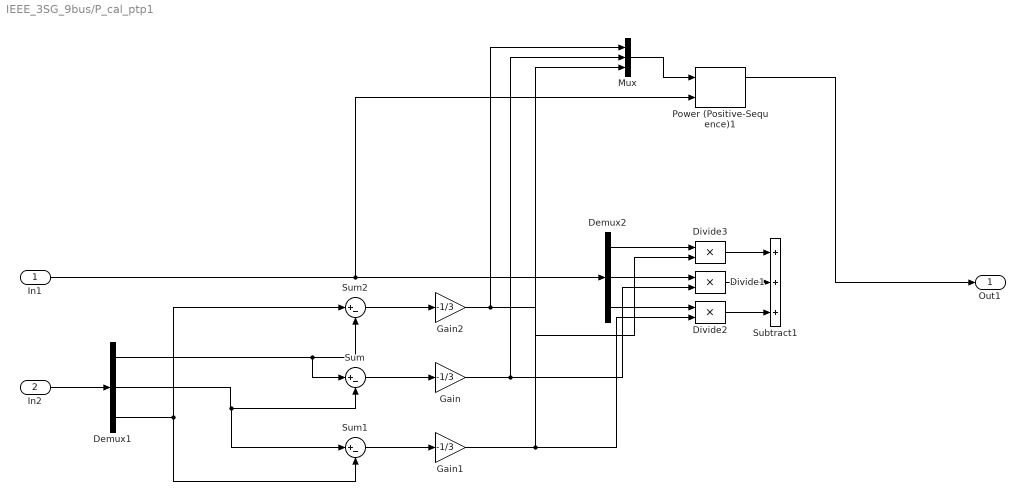
== system IEEE_3SG_9bus/P_cal_ptp1 ==
  In1 : Inport
  In2 : Inport  Port=2
  Demux1 : Demux  Outputs=3
  Demux2 : Demux  Outputs=3
  Divide1 : Product  Inputs=**
  Divide2 : Product  Inputs=**
  Divide3 : Product  Inputs=**
  Gain : Gain  Gain=-1/3
  Gain1 : Gain  Gain=-1/3
  Gain2 : Gain  Gain=-1/3
  Mux : Mux  Inputs=3
  Power (Positive-Sequence)1 : spsPowerPositiveSequenceLib/Power (Positive-Sequence)  Freq=60  Vinit=[0, 0]  Iinit=[0, 0]  Ts=1e-4
  Subtract1 : Sum  Inputs=+++
  Sum : Sum  Inputs=|+-
  Sum1 : Sum  Inputs=|+-
  Sum2 : Sum  Inputs=|+-
  Out1 : Outport
  wires:
  Sum2/1 -> Gain2/1
  Demux1/3 -> Sum2/1, Sum1/2
  Demux1/1 -> Sum2/2, Sum/1
  Demux1/2 -> Sum1/1, Sum/2
  Demux2/2 -> Divide1/1
  Gain1/1 -> Divide2/2, Mux/3
  Divide1/1 -> Subtract1/2
  Divide3/1 -> Subtract1/1
  Sum1/1 -> Gain1/1
  In1/1 -> Power (Positive-Sequence)1/2, Demux2/1
  Divide2/1 -> Subtract1/3
  Demux2/3 -> Divide2/1
  Demux2/1 -> Divide3/1
  Gain/1 -> Mux/2, Divide1/2
  Sum/1 -> Gain/1
  Gain2/1 -> Mux/1, Divide3/2
  In2/1 -> Demux1/1
  Power (Positive-Sequence)1/1 -> Out1/1
  Mux/1 -> Power (Positive-Sequence)1/1

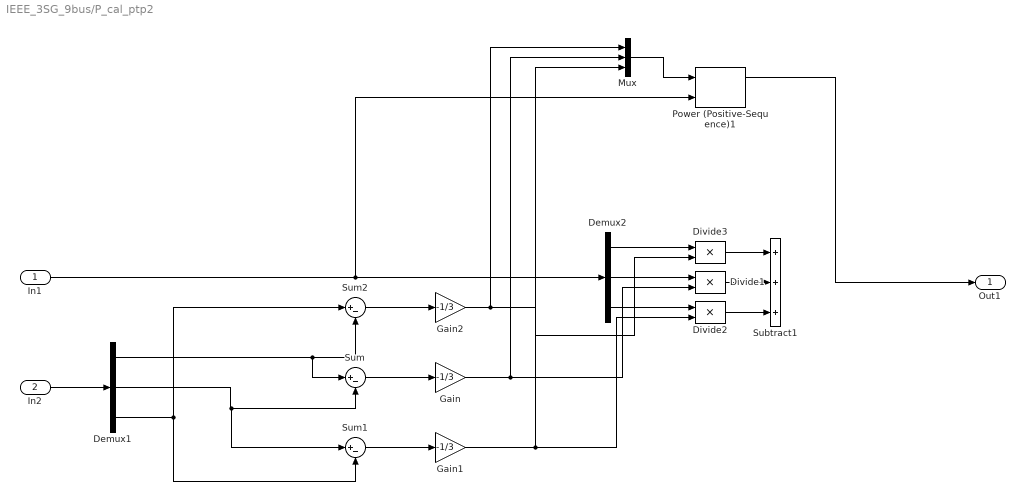
== system IEEE_3SG_9bus/P_cal_ptp2 ==
  In1 : Inport
  In2 : Inport  Port=2
  Demux1 : Demux  Outputs=3
  Demux2 : Demux  Outputs=3
  Divide1 : Product  Inputs=**
  Divide2 : Product  Inputs=**
  Divide3 : Product  Inputs=**
  Gain : Gain  Gain=-1/3
  Gain1 : Gain  Gain=-1/3
  Gain2 : Gain  Gain=-1/3
  Mux : Mux  Inputs=3
  Power (Positive-Sequence)1 : spsPowerPositiveSequenceLib/Power (Positive-Sequence)  Freq=60  Vinit=[0, 0]  Iinit=[0, 0]  Ts=1e-4
  Subtract1 : Sum  Inputs=+++
  Sum : Sum  Inputs=|+-
  Sum1 : Sum  Inputs=|+-
  Sum2 : Sum  Inputs=|+-
  Out1 : Outport
  wires:
  Sum2/1 -> Gain2/1
  Demux1/3 -> Sum2/1, Sum1/2
  Demux1/1 -> Sum2/2, Sum/1
  Demux1/2 -> Sum1/1, Sum/2
  Demux2/2 -> Divide1/1
  Gain1/1 -> Divide2/2, Mux/3
  Divide1/1 -> Subtract1/2
  Divide3/1 -> Subtract1/1
  Sum1/1 -> Gain1/1
  In1/1 -> Power (Positive-Sequence)1/2, Demux2/1
  Divide2/1 -> Subtract1/3
  Demux2/3 -> Divide2/1
  Demux2/1 -> Divide3/1
  Gain/1 -> Mux/2, Divide1/2
  Sum/1 -> Gain/1
  Gain2/1 -> Mux/1, Divide3/2
  In2/1 -> Demux1/1
  Power (Positive-Sequence)1/1 -> Out1/1
  Mux/1 -> Power (Positive-Sequence)1/1

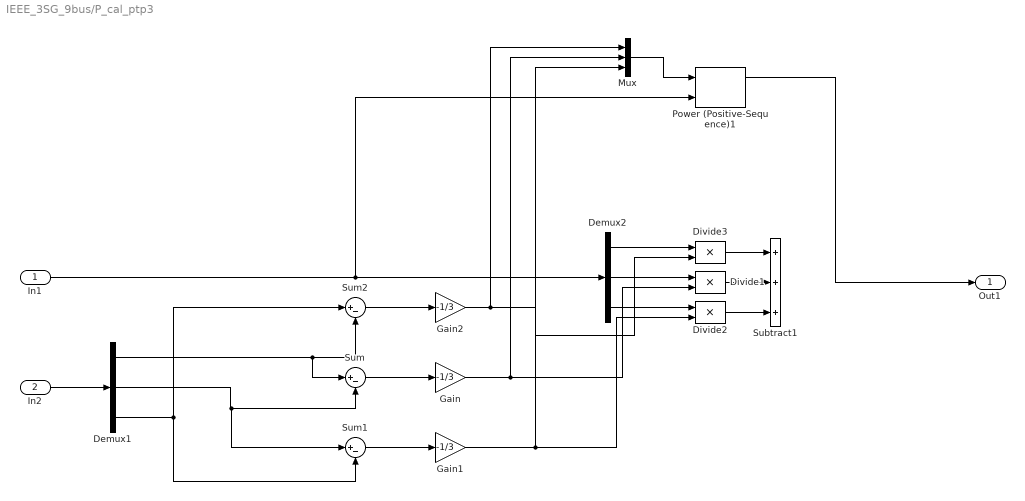
== system IEEE_3SG_9bus/P_cal_ptp3 ==
  In1 : Inport
  In2 : Inport  Port=2
  Demux1 : Demux  Outputs=3
  Demux2 : Demux  Outputs=3
  Divide1 : Product  Inputs=**
  Divide2 : Product  Inputs=**
  Divide3 : Product  Inputs=**
  Gain : Gain  Gain=-1/3
  Gain1 : Gain  Gain=-1/3
  Gain2 : Gain  Gain=-1/3
  Mux : Mux  Inputs=3
  Power (Positive-Sequence)1 : spsPowerPositiveSequenceLib/Power (Positive-Sequence)  Freq=60  Vinit=[0, 0]  Iinit=[0, 0]  Ts=1e-4
  Subtract1 : Sum  Inputs=+++
  Sum : Sum  Inputs=|+-
  Sum1 : Sum  Inputs=|+-
  Sum2 : Sum  Inputs=|+-
  Out1 : Outport
  wires:
  Sum2/1 -> Gain2/1
  Demux1/3 -> Sum2/1, Sum1/2
  Demux1/1 -> Sum2/2, Sum/1
  Demux1/2 -> Sum1/1, Sum/2
  Demux2/2 -> Divide1/1
  Gain1/1 -> Divide2/2, Mux/3
  Divide1/1 -> Subtract1/2
  Divide3/1 -> Subtract1/1
  Sum1/1 -> Gain1/1
  In1/1 -> Power (Positive-Sequence)1/2, Demux2/1
  Divide2/1 -> Subtract1/3
  Demux2/3 -> Divide2/1
  Demux2/1 -> Divide3/1
  Gain/1 -> Mux/2, Divide1/2
  Sum/1 -> Gain/1
  Gain2/1 -> Mux/1, Divide3/2
  In2/1 -> Demux1/1
  Power (Positive-Sequence)1/1 -> Out1/1
  Mux/1 -> Power (Positive-Sequence)1/1
